simulink model "GFLIB_ControllerPIrAW_BAM"  (Simulink 9.3)
settings: Solver=VariableStepAuto  StartTime=0.0  StopTime=10.0  RelTol=1e-3
settings Model: Creator=nxa18952  LastModifiedBy=nxa18952
settings DataIOCC: SaveFormat=Dataset  SignalLoggingSaveFormat=Dataset  ReturnWorkspaceOutputs=on
settings OptimizationCC: LifeSpan=auto
settings DebuggingCC: UnderspecifiedInitializationDetection=Simplified  MergeDetectMultiDrivingBlocksExec=error  FcnCallInpInsideContextMsg=error  SFUnexpectedBacktrackingDiag=error  SFNoUnconditionalDefaultTransitionDiag=error  SFExecutionAtInitializationDiag=warning  ArithmeticOperatorsInVariantConditions=error
settings HardwareCC: ProdBitPerPointer=64  ProdBitPerSizeT=64  ProdBitPerPtrDiffT=64  ProdLargestAtomicFloat=Float  ProdIntDivRoundTo=Zero  ProdEndianess=LittleEndian  ProdWordSize=64  ProdHWDeviceType=Intel->x86-64 (Windows64)
settings ModelReferenceCC: PropagateSignalLabelsOutOfModel=on
settings SFSimCC: SimUseLocalCustomCode=on
settings RTWCC: RTWUseLocalCustomCode=on
settings CodeAppCC: StateflowObjectComments=off
settings GRTTargetCC: TargetLangStandard=C99 (ISO)  CombineOutputUpdateFcns=on  GRTInterface=off
settings ConfigComp: CovMetricSettings=dwe  CovHtmlReporting=off  CovSaveCumulativeToWorkspaceVar=off  CovSaveSingleToWorkspaceVar=off  CovExternalEMLEnable=on

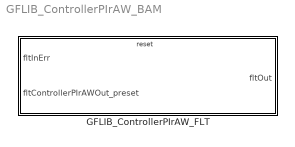
== system GFLIB_ControllerPIrAW_BAM ==
  GFLIB_ControllerPIrAW_FLT : Subsystem  TreatAsAtomicUnit=on  mask(GFLIB_ControllerPIrAW_FLT){showStates=Hide (faster execution), resetStatesEnable=Pre-set according to the first set of inputs after reset, fltUpperLimit=0, fltLowerLimit=0, fltCC1sc=0, fltCC2sc=0}
      mask prompts: showStates "Show internal states"; resetStatesEnable "Internal state after reset"; fltUpperLimit "fltUpperLimit (Upper Limit of the controller)"; fltLowerLimit "fltLowerLimit (Lower Limit of the controller)"; fltCC1sc "fltCC1sc (CC1 coefficient)"; fltCC2sc "fltCC2sc (CC2 coefficient)"
      mask help: Recurrent form PI controller with anti-windup in single precision floating-point implementation. This block supports re-initialization of the internal state during simulation. If the block is reset, the controller's output will be aligned with the input fltControllerPIrAWOut_preset. Refer to the AMMCLIB User's Guide for further details.
      mask init:
      | if ~evalin('base','exist(''tS8'',''var'')')
      |   if (2 ~= exist('SWLIBS_Typedefs.mat','file'))
      |       error('File SWLIBS_Typedefs.mat is not on the Matlab path. Please add the AMMCLIB "bam" folder in the Matlab Search Path.');
      |   else
      |       evalin('base', 'load(''SWLIBS_Typedefs.mat'')');
      |   end
      | end
      | if showStates == 1
      |     % hidden state variables
      |     if strcmp(get_param([gcb '/fltUpperLimit'], 'BlockType'), 'Inport')
      |         posblk = get_param(gcb, 'Position');
      | 
      |         pos = get_param(    [gcb, '/fltUpperLimit'], 'Position');
      |         orient = get_param( [gcb, '/fltUpperLimit'], 'Orientation');
      |         delete_block(       [gcb, '/fltUpperLimit']);
      |         add_block('built-in/Ground', [gcb, '/fltUpperLimit'], 'Position', pos, 'Orientation', orient);
      | 
      |         pos = get_param(    [gcb, '/fltLowerLimit'], 'Position');
      |         orient = get_param( [gcb, '/fltLowerLimit'], 'Orientation');
      |         delete_block(       [gcb, '/fltLowerLimit']);
      |         add_block('built-in/Ground', [gcb, '/fltLowerLimit'], 'Position', pos, 'Orientation', orient);
      | 
      |         pos = get_param(    [gcb, '/fltAcc'], 'Position');
      |         orient = get_param( [gcb, '/fltAcc'], 'Orientation');
      |         delete_block(       [gcb, '/fltAcc']);
      |         add_block('built-in/Ground', [gcb, '/fltAcc'], 'Position', pos, 'Orientation', orient);
      | 
      |         pos = get_param(    [gcb, '/fltInErrK1'], 'Position');
      |         orient = get_param( [gcb, '/fltInErrK1'], 'Orientation');
      |         delete_block(       [gcb, '/fltInErrK1']);
      |         add_block('built-in/Ground', [gcb, '/fltInErrK1'], 'Position', pos, 'Orientation', orient);
      | 
      |         pos = get_param(    [gcb, '/fltCC1sc'], 'Position');
      |         orient = get_param( [gcb, '/fltCC1sc'], 'Orientation');
      |         delete_block(       [gcb, '/fltCC1sc']);
      |         add_block('built-in/Ground', [gcb, '/fltCC1sc'], 'Position', pos, 'Orientation', orient);
      | 
      |         pos = get_param(    [gcb, '/fltCC2sc'], 'Position');
      |         orient = get_param( [gcb, '/fltCC2sc'], 'Orientation');
      |         delete_block(       [gcb, '/fltCC2sc']);
      |         add_block('built-in/Ground', [gcb, '/fltCC2sc'], 'Position', pos, 'Orientation', orient);
      | 
      | 
      |         pos = get_param(    [gcb '/fltAcc_Out'], 'Position');
      |         orient = get_param( [gcb '/fltAcc_Out'], 'Orientation');
      |         delete_block(       [gcb '/fltAcc_Out']);
      |         add_block('built-in/Terminator', [gcb '/fltAcc_Out'], 'Position', pos, 'Orientation', orient);
      | 
      |         pos = get_param(    [gcb '/fltInErrK1_Out'], 'Position');
      |         orient = get_param( [gcb '/fltInErrK1_Out'], 'Orientation');
      |         delete_block(       [gcb '/fltInErrK1_Out']);
      |         add_block('built-in/Terminator', [gcb '/fltInErrK1_Out'], 'Position', pos, 'Orientation', orient);
      | 
      | 
      |         set_param([gcb '/fltInErr'], 'Port', '1');
      |         set_param([gcb '/fltControllerPIrAWOut_preset'], 'Port', '2');
      | 
      |         set_param([gcb '/fltOut'], 'Port', '1');
      | 
      |         set_param(gcb,'MaskEnables',{'on','on','on','on','on','on'});
      | 
      |         if (posblk(4) - posblk(2)) > 75
      |           height = 75;
      |           set_param(gcb,'Position',[posblk(1), posblk(2), posblk(3), posblk(2)+height])
      |         end
      |     end
      | else
      |     % shown state variables
      |     if strcmp(get_param([gcb '/fltUpperLimit'], 'BlockType'), 'Ground')
      |         posblk = get_param(gcb, 'Position');
      | 
      |         pos = get_param(    [gcb, '/fltUpperLimit'], 'Position');
      |         orient = get_param( [gcb, '/fltUpperLimit'], 'Orientation');
      |         delete_block(       [gcb, '/fltUpperLimit']);
      |         add_block('built-in/Inport', [gcb, '/fltUpperLimit'], 'Position', pos, 'Orientation', orient, 'OutDataTypeStr', 'single');
      | 
      |         pos = get_param(    [gcb, '/fltLowerLimit'], 'Position');
      |         orient = get_param( [gcb, '/fltLowerLimit'], 'Orientation');
      |         delete_block(       [gcb, '/fltLowerLimit']);
      |         add_block('built-in/Inport', [gcb, '/fltLowerLimit'], 'Position', pos, 'Orientation', orient, 'OutDataTypeStr', 'single');
      | 
      |         pos = get_param(    [gcb, '/fltAcc'], 'Position');
      |         orient = get_param( [gcb, '/fltAcc'], 'Orientation');
      |         delete_block(       [gcb, '/fltAcc']);
      |         add_block('built-in/Inport', [gcb, '/fltAcc'], 'Position', pos, 'Orientation', orient, 'OutDataTypeStr', 'single');
      | 
      |         pos = get_param(    [gcb, '/fltInErrK1'], 'Position');
      |         orient = get_param( [gcb, '/fltInErrK1'], 'Orientation');
      |         delete_block(       [gcb, '/fltInErrK1']);
      |         add_block('built-in/Inport', [gcb, '/fltInErrK1'], 'Position', pos, 'Orientation', orient, 'OutDataTypeStr', 'single');
      | 
      |         pos = get_param(    [gcb, '/fltCC1sc'], 'Position');
      |         orient = get_param( [gcb, '/fltCC1sc'], 'Orientation');
      |         delete_block(       [gcb, '/fltCC1sc']);
      |         add_block('built-in/Inport', [gcb, '/fltCC1sc'], 'Position', pos, 'Orientation', orient, 'OutDataTypeStr', 'single');
      | 
      |         pos = get_param(    [gcb, '/fltCC2sc'], 'Position');
      |         orient = get_param( [gcb, '/fltCC2sc'], 'Orientation');
      |         delete_block(       [gcb, '/fltCC2sc']);
      |         add_block('built-in/Inport', [gcb, '/fltCC2sc'], 'Position', pos, 'Orientation', orient, 'OutDataTypeStr', 'single');
      | 
      | 
      |         pos = get_param(    [gcb '/fltAcc_Out'], 'Position');
      |         orient = get_param( [gcb '/fltAcc_Out'], 'Orientation');
      |         delete_block(       [gcb '/fltAcc_Out']);
      |         add_block('built-in/Outport', [gcb '/fltAcc_Out'], 'Position', pos, 'Orientation', orient);
      | 
      |         pos = get_param(    [gcb '/fltInErrK1_Out'], 'Position');
      |         orient = get_param( [gcb '/fltInErrK1_Out'], 'Orientation');
      |         delete_block(       [gcb '/fltInErrK1_Out']);
      |         add_block('built-in/Outport', [gcb '/fltInErrK1_Out'], 'Position', pos, 'Orientation', orient);
      | 
      | 
      |         set_param([gcb '/fltInErr'], 'Port', '1');
      |         set_param([gcb '/fltControllerPIrAWOut_preset'], 'Port', '2');
      |         set_param([gcb '/fltUpperLimit'], 'Port', '3');
      |         set_param([gcb '/fltLowerLimit'], 'Port', '4');
      |         set_param([gcb '/fltAcc'], 'Port', '5');
      |         set_param([gcb '/fltInErrK1'], 'Port', '6');
      |         set_param([gcb '/fltCC1sc'], 'Port', '7');
      |         set_param([gcb '/fltCC2sc'], 'Port', '8');
      | 
      |         set_param([gcb '/fltOut'], 'Port', '1');
      |         set_param([gcb '/fltAcc_Out'], 'Port', '2');
      |         set_param([gcb '/fltInErrK1_Out'], 'Port', '3');
      | 
      |         set_param(gcb,'MaskEnables',{'on','on','off','off','off','off'});
      | 
      |         if (posblk(4) - posblk(2)) < 225
      |           height = 225;
      |           set_param(gcb,'Position',[posblk(1), posblk(2), posblk(3), posblk(2)+height])
      |         end
      |     end
      | end
      settings: RTWSystemCode=Inline
      mask TypeOptions showStates: Hide (faster execution) | Show (allows debugging; connect feedback loops manually)
      mask Callback showStates:
      | maskStr = get_param(gcb,'showStates');
      | if strcmp(maskStr,'Hide (faster execution)'),
      |     set_param(gcb,'MaskEnables',{'on','on','on','on','on','on'});
      | else
      |     set_param(gcb,'MaskEnables',{'on','on','off','off','off','off'});
      | end
      mask TypeOptions resetStatesEnable: Pre-set according to the first set of inputs after reset | Clear to zero
      mask Display:
      | color('black');
      | pos = get_param(gcb, 'Position');
      | width = pos(3) - pos(1);
      | height = pos(4) - pos(2);
      | tX=width/2;
      | tY=height - 25;
      | color('black');
      | text(tX,tY, 'GFLIB_ControllerPIrAW_FLT', 'horizontalAlignment', 'center');
      | if showStates == 2
      |   color('red');
      |   text(tX,tY - 20, ['debugging mode' char(13) char(10) '(limited performance)'], 'horizontalAlignment', 'center');
      | end

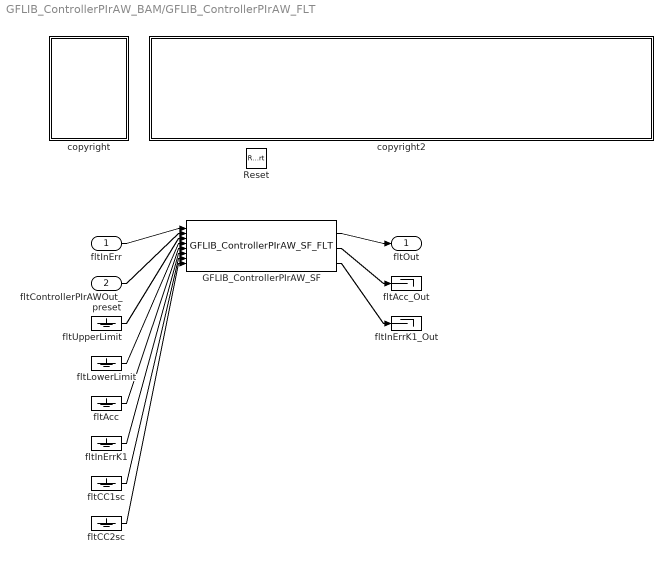
== system GFLIB_ControllerPIrAW_BAM/GFLIB_ControllerPIrAW_FLT ==
  fltInErr : Inport  OutDataTypeStr=single
  fltControllerPIrAWOut_preset : Inport  Port=2  OutDataTypeStr=single
  Reset : ResetPort  DisableCoverage=on
  GFLIB_ControllerPIrAW_SF : S-Function  FunctionName=GFLIB_ControllerPIrAW_SF_FLT  Parameters=showStates,resetStatesEnable,fltUpperLimit,fltLowerLimit,fltCC1sc,fltCC2sc  SFunctionDeploymentMode=off  EnableBusSupport=off
  copyright : Subsystem
      mask Display: text(10,90,'FILE:');text(10,75,'DESRIPTION:');text(10,60,'COPYRIGHT:');text(10,45,'VERSION:');text(10,30,'DATE:')
  copyright2 : Subsystem
      mask Display: text(10,90,'GFLIB_ControllerPIrAW_BAM_FLT.mdl');text(10,75,'Recurrent form PI controller with anti-windup.');text(10,60,'NXP 2020');text(10,45,'1.0');text(10,30,'28-Mar-2020');
  fltAcc : Ground
  fltAcc_Out : Terminator
  fltCC1sc : Ground
  fltCC2sc : Ground
  fltInErrK1 : Ground
  fltInErrK1_Out : Terminator
  fltLowerLimit : Ground
  fltUpperLimit : Ground
  fltOut : Outport
  wires:
  fltInErr/1 -> GFLIB_ControllerPIrAW_SF/1
  fltControllerPIrAWOut_preset/1 -> GFLIB_ControllerPIrAW_SF/2
  fltUpperLimit/1 -> GFLIB_ControllerPIrAW_SF/3
  fltLowerLimit/1 -> GFLIB_ControllerPIrAW_SF/4
  fltAcc/1 -> GFLIB_ControllerPIrAW_SF/5
  fltInErrK1/1 -> GFLIB_ControllerPIrAW_SF/6
  fltCC1sc/1 -> GFLIB_ControllerPIrAW_SF/7
  fltCC2sc/1 -> GFLIB_ControllerPIrAW_SF/8
  GFLIB_ControllerPIrAW_SF/1 -> fltOut/1
  GFLIB_ControllerPIrAW_SF/2 -> fltAcc_Out/1
  GFLIB_ControllerPIrAW_SF/3 -> fltInErrK1_Out/1

== system GFLIB_ControllerPIrAW_BAM/GFLIB_ControllerPIrAW_FLT/copyright ==

== system GFLIB_ControllerPIrAW_BAM/GFLIB_ControllerPIrAW_FLT/copyright2 ==
